simulink model "shapesim_lite"  (R2022a)
settings: Solver=ode3  StartTime=s.start_time  StopTime=s.stop_time  FixedStep=s.step_time  MaxStep=step_time*1000  MinStep=step_time/10  RelTol=1e-3
values from neighbouring files (symbols this model uses):
  Actuators = nstxu_Actuators()    [setup_nstxu.m]    (also in startup.m)
  Tokamak = nstxu_Tokamak(s)    [setup_nstxu.m]    (also in startup.m)
undefined symbols (not defined in the file or in its folder): curdir, iy, latency, opt, slewratemax, slewratemin, tbd, vbd, vmax, vmin
libraries: cstblocks x1, simulink x1, toksim_generic x1
settings Model: Creator=welander  LastModifiedBy=jwai
settings SolverCC: InitialStep=step_time  MaxConsecutiveMinStep=3  AlgebraicLoopSolver=TrustRegion
settings DataIOCC: SaveFormat=Array  SaveOutput=off  SignalLogging=off  DSMLogging=off  SaveTime=off  ReturnWorkspaceOutputs=off
settings OptimizationCC: BlockReduction=off  BooleanDataType=off  LifeSpan=inf
settings DebuggingCC: SaveWithParameterizedLinksMsg=none  UnderspecifiedInitializationDetection=Classic  MergeDetectMultiDrivingBlocksExec=none  SignalResolutionControl=TryResolveAllWithWarning  UnconnectedInputMsg=warning  UnconnectedOutputMsg=warning  UnconnectedLineMsg=warning  SFUnexpectedBacktrackingDiag=warning  SFNoUnconditionalDefaultTransitionDiag=warning  SFExecutionAtInitializationDiag=none  SFMachineParentedDataDiag=warning  ArithmeticOperatorsInVariantConditions=warning
settings HardwareCC: ProdBitPerPointer=32  ProdBitPerSizeT=32  ProdBitPerPtrDiffT=32  ProdLargestAtomicFloat=None  ProdIntDivRoundTo=Undefined  ProdEndianess=Unspecified  ProdWordSize=32  ProdHWDeviceType=32-bit Generic  TargetUnknown=on
settings ModelReferenceCC: PropagateSignalLabelsOutOfModel=off
settings SFSimCC: SimUseLocalCustomCode=off  CustomCodeUndefinedFunction=UseInterfaceOnly
settings RTWCC: RTWUseLocalCustomCode=off  DLArmComputeVersion=19.05
settings CodeAppCC: StateflowObjectComments=on
settings GRTTargetCC: TargetLangStandard=C89/C90 (ANSI)
settings ConfigComp: CovMetricSettings=dw  CovSaveCumulativeToWorkspaceVar=on  CovSaveSingleToWorkspaceVar=on  CovExternalEMLEnable=off  CovSFcnEnable=off

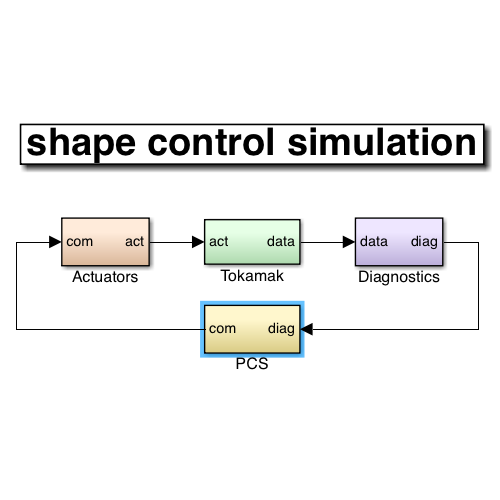
[thumbnail: Simulink's stored preview of the top-level diagram]
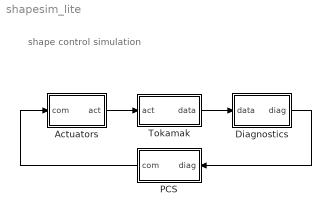
== system shapesim_lite ==
  note: shape control simulation
  Actuators : Subsystem
  Diagnostics : Subsystem
  PCS : Subsystem
  Tokamak : Subsystem
  wires:
  Diagnostics/1(diag) -> PCS/1(diag)
  Actuators/1(act) -> Tokamak/1(act)
  Tokamak/1(data) -> Diagnostics/1(data)
  PCS/1(com) -> Actuators/1(com)

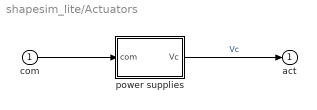
== system shapesim_lite/Actuators ==
  com : Inport
  power supplies : Subsystem  Description=Model of power supplies for circuits with coils. The outputs are applied voltages on circuits of coils and are therefore boundary conditions at the coils.  mask{config=Actuators.PS}
      mask init:
      | if isstruct(config)
      |     struct_to_ws(config);
      | end
  act : Outport
  wires:
  power supplies/1(Vc) -> act/1  "Vc"
  com/1 -> power supplies/1(com)

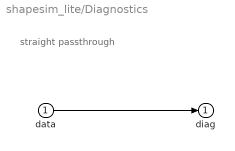
== system shapesim_lite/Diagnostics ==
  note: straight passthrough
  data : Inport
  diag : Outport
  wires:
  data/1 -> diag/1

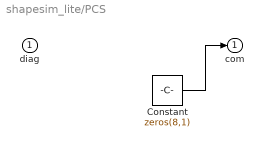
== system shapesim_lite/PCS ==
  diag : Inport
  Constant : Constant  Value=zeros(8,1)
  com : Outport
  wires:
  Constant/1 -> com/1

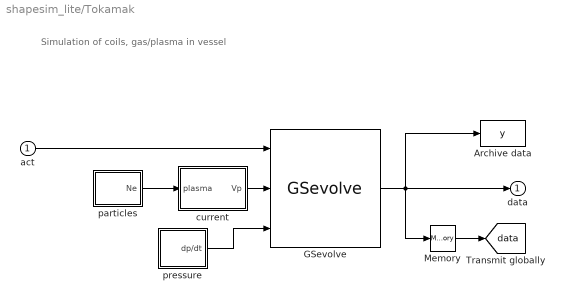
== system shapesim_lite/Tokamak ==
  note: Simulation of coils, gas/plasma in vessel
  act : Inport
  Archive data : ToWorkspace  VariableName=y  SaveFormat=Timeseries  SampleTime=-1
      settings: Decimation=s.decimation
  GSevolve : toksim_generic/Tokamak_Plasma_Modules/GSevolve  Tag=d3d/Tokamak/GSevolve  Description=PCSSP module  config=Tokamak.c  init=Tokamak.e
      settings: SourceProductName=TokSys
  Memory : Memory  InitialCondition=Tokamak.yinit
  current : Subsystem  mask{jconfig=Tokamak.current}
      mask prompts: jconfig "Current config"
      mask init:
      | if isstruct(jconfig)
      |     struct_to_ws(jconfig);
      | end
  particles : Subsystem  mask{config=Tokamak.particles}
      mask prompts: config "Settings"
      mask init:
      | if isstruct(config)
      |     struct_to_ws(config);
      | end
      | 
      | % For proper initialization of ionization:
      | clear ionization
  pressure : Subsystem  mask{pressure=Tokamak.pressure}
      mask prompts: pressure "Configuration of pressure model"
      mask init:
      | if isstruct(pressure)
      |     struct_to_ws(pressure);
      | end
  data : Outport
  tag scope: data=global
  wires:
  GSevolve/1 -> Archive data/1, data/1, Memory/1
  act/1 -> GSevolve/1
  current/1(Vp) -> GSevolve/2
  particles/1(Ne) -> current/1(plasma)
  pressure/1(dp/dt) -> GSevolve/3
  Memory/1 -> [data]

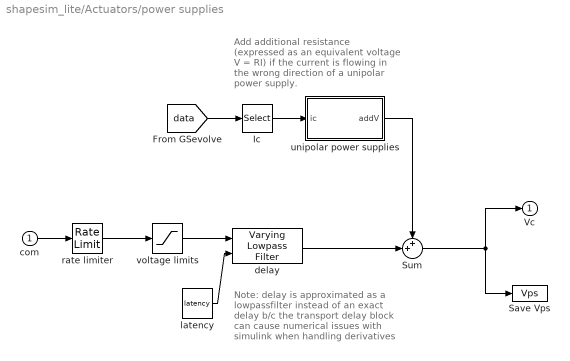
== system shapesim_lite/Actuators/power supplies ==
  note: Note: delay is approximated as a lowpassfilter instead of an exact delay b/c the transport delay block can cause numerical issues with simulink when handling derivatives
  note: Add additional resistance (expressed as an equivalent voltage V = RI) if the current is flowing in the wrong direction of a unipolar power supply.
  com : Inport
  Ic : Selector  IndexOptions=Index vector (dialog)  Indices=c.iy.ic  OutputSizes=1
  Save Vps : ToWorkspace  VariableName=Vps  SaveFormat=Timeseries  SampleTime=-1
      settings: Decimation=s.decimation
  Sum : Sum  Inputs=++|
  delay : cstblocks/Linear Parameter Varying/Varying Lowpass Filter  N=1
  latency : Constant  Value=latency
  rate limiter : RateLimiter  RisingSlewLimit=slewratemax  FallingSlewLimit=slewratemin
  unipolar power supplies : Subsystem
  voltage limits : Saturate  UpperLimit=vmax  LowerLimit=vmin  ZeroCross=off
  Vc : Outport
  wires:
  rate limiter/1 -> voltage limits/1
  [data] -> Ic/1
  com/1 -> rate limiter/1
  Sum/1 -> Save Vps/1, Vc/1
  Ic/1 -> unipolar power supplies/1(ic)
  unipolar power supplies/1(addV) -> Sum/1
  voltage limits/1 -> delay/1
  delay/1 -> Sum/2
  latency/1 -> delay/2

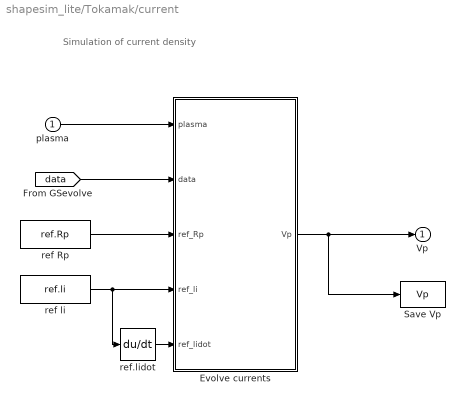
== system shapesim_lite/Tokamak/current ==
  note: Simulation of current density
  plasma : Inport
  Evolve currents : MATLAB Function  TreatAsAtomicUnit=on
  Save Vp : ToWorkspace  VariableName=Vp  SaveFormat=Timeseries  SampleTime=-1
      settings: Decimation=s.decimation
  ref Rp : FromWorkspace  VariableName=ref.Rp  OutputAfterFinalValue=Holding final value
  ref li : FromWorkspace  VariableName=ref.li  OutputAfterFinalValue=Holding final value
  ref.lidot : Derivative
  Vp : Outport
  wires:
  plasma/1 -> Evolve currents/1(plasma)
  [data] -> Evolve currents/2(data)
  Evolve currents/1(Vp) -> Save Vp/1, Vp/1
  ref Rp/1 -> Evolve currents/3(ref_Rp)
  ref li/1 -> ref.lidot/1, Evolve currents/4(ref_li)
  ref.lidot/1 -> Evolve currents/5(ref_lidot)

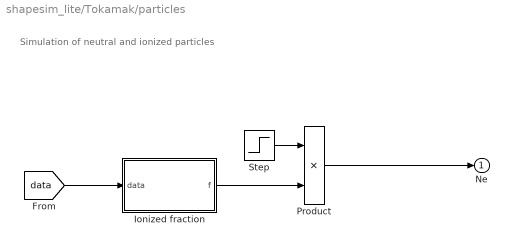
== system shapesim_lite/Tokamak/particles ==
  note: Simulation of neutral and ionized particles
  Ionized fraction : MATLAB Function  TreatAsAtomicUnit=on
  Product : Product
  Step : Step  Time=tbd  SampleTime=0
  Ne : Outport
  wires:
  Ionized fraction/1(f) -> Product/2
  Product/1 -> Ne/1
  [data] -> Ionized fraction/1(data)
  Step/1 -> Product/1

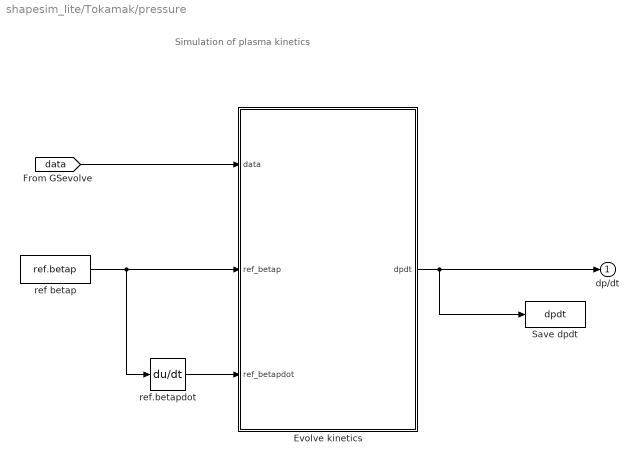
== system shapesim_lite/Tokamak/pressure ==
  note: Simulation of plasma kinetics
  Evolve kinetics : MATLAB Function  TreatAsAtomicUnit=on
  Save dpdt : ToWorkspace  VariableName=dpdt  SaveFormat=Timeseries  SampleTime=-1
      settings: Decimation=s.decimation
  ref betap : FromWorkspace  VariableName=ref.betap  OutputAfterFinalValue=Holding final value
  ref.betapdot : Derivative
  dp/dt : Outport
  wires:
  [data] -> Evolve kinetics/1(data)
  ref betap/1 -> Evolve kinetics/2(ref_betap), ref.betapdot/1
  ref.betapdot/1 -> Evolve kinetics/3(ref_betapdot)
  Evolve kinetics/1(dpdt) -> Save dpdt/1, dp/dt/1

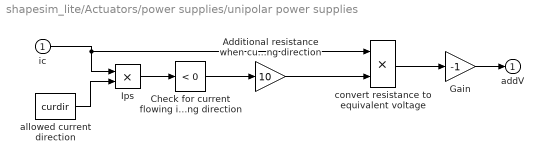
== system shapesim_lite/Actuators/power supplies/unipolar power supplies ==
  ic : Inport
  Additional resistance when current in wrong direction : Gain  Gain=10
  Check for current flowing in the wrong direction : simulink/Logic and Bit Operations/Compare To Constant  relop=<  const=0  OutDataTypeStr=boolean
  Gain : Gain  Gain=-1
  Ips : Product  Inputs=**
  allowed current direction : Constant  Value=curdir
  convert resistance to equivalent voltage : Product
  addV : Outport
  wires:
  ic/1 -> convert resistance to equivalent voltage/1, Ips/1
  allowed current direction/1 -> Ips/2
  Ips/1 -> Check for current flowing in the wrong direction/1
  Check for current flowing in the wrong direction/1 -> Additional resistance when current in wrong direction/1
  Additional resistance when current in wrong direction/1 -> convert resistance to equivalent voltage/2
  convert resistance to equivalent voltage/1 -> Gain/1
  Gain/1 -> addV/1

== matlab function shapesim_lite/Tokamak/particles/Ionized fraction ==
  data: data input; f output; iy parameter; vbd parameter
function f = ionization(data, iy, vbd)

% Remember previous fraction of ionization
persistent fprev
if isempty(fprev)
    fprev = nan;
end

% 0 = no jphi, 1 = faeq, 2 = GS, 3 = terminating
gsphase = data(iy.gsphase);

if isnan(fprev)
    % Initialize ionization
    if gsphase == 0 | gsphase == 3
        f = 0;
    else
        f = 1;
    end
else
    % fprev exists
    if gsphase == 3
        % Neutralize!
        f = 0;
    elseif fprev > 0
        f = fprev;
    else
        % Breakdown?
        ibd = abs(data(iy.vdp)) > vbd;
        if any(ibd)
            % Check connection length for points with enough field
            % Then decide f (skipping connection length test for now)
            f = 1;
        else
            % Insufficient E-field for breakdown
            f = 0;
        end
    end
end


fprev = f;

== matlab function shapesim_lite/Tokamak/pressure/Evolve kinetics ==
  data: data input; ref_betap input; ref_betapdot input; iy parameter; dpdt output size=opt.ndpdt; opt parameter
function  dpdt = kinetics(data, ref_betap, ref_betapdot, iy, opt)

betap = data(iy.betap);
gsphase = data(iy.gsphase);


dpdt = zeros(opt.ndpdt,1);
if gsphase == 0
    % Sending zeros
elseif gsphase == 1
    % Sending zeros
elseif gsphase == 2
    dpdt = ref_betapdot + opt.P*(ref_betap-betap);
else
    % Sending zeros during termination
end

== matlab function shapesim_lite/Tokamak/current/Evolve currents ==
  data ref_Rp settings: description=Preprogrammed outputs
  data: plasma input; data input; ref_Rp input; ref_li input; ref_lidot input; Vp output size=opt.nVp; iy parameter; opt parameter
function Vp = current(plasma, data, ref_Rp, ref_li, ref_lidot, iy, opt)

%%%%%%%%%%%%%%%%%%%%%%%%%%%%%%%%%%%%%%%%%%%%%%%%%%%%%%%%%%%%%%%%%%%%%%%%%%%
%
%  USAGE:   [jboot, eta] = bootstrap(data, kin, ref, idx)
%
%  PURPOSE: Calculate bootstrap current and related quantities
%
%  INPUTS: data = vector of GSevolve outputs containing profile information
%             psip,   poloidal flux on flux surfaces [Wb]
%             rsurf,  radial center of flux surfaces [m]
%             aminor, minor radius of flux surfaces [m]
%             fpol,   fpol = 2e-7*enclosed poloidal current [Wb]
%             pres,   pressure [Pa]
%             q,      safety factor
%             ft,     fraction trapped particles in collisionless limit
%             Babs,   Surface-averaged B field magnitude
%          kin = vector pressure outputs containing profile information
%             pe, electron pressure [N/m2]
%             ne, electron density [m-3]
%             pi, ion pressure [N/m2]
%             Z, Zeff proxy
%
%  OUTPUTS: jboot = <jbs*B>/<B>
%           eta = neoclassical resistivity
%
%  Calculations are done with formulas found in:
%  Neoclassical conductivity and bootstrap current formulas for general
%  axisymmetric equilibria and arbitrary collisionality regime,
%  Sauter et al, Physics of Plasmas 6, 2834 (1999) & erratum 9, 5140 (2002)
%
%  RESTRICTIONS: Potato orbits near axis are not considered
%                Approximate treatment for multiple ion species
	
	
%  WRITTEN BY: Anders Welander ON 2020-07-22 from bootstrap.m in TokSys
%
%  MODIFICATION HISTORY:				
%	
%%%%%%%%%%%%%%%%%%%%%%%%%%%%%%%%%%%%%%%%%%%%%%%%%%%%%%%%%%%%%%%%%%%%%%%%%%%


Ip = data(iy.cpasma);
li = data(iy.li);
gsphase = data(iy.gsphase);
Rp = ref_Rp;
Vp = zeros(opt.nVp,1);


if gsphase == 0
  if plasma
    Vp(1) = 10;
  end
elseif gsphase == 1
  Vp(1) = -Rp*Ip;
elseif gsphase == 2
  if opt.evolve_option == 1
    Vp(1) = -Rp*Ip;
    Vp(2) = ref_lidot + opt.P*(ref_li-li);
  end
else
  % Sending zeros during termination
end
